simulink model "ex_mass_spring_damper_appdemo"  (R2024b)
settings: Solver=VariableStepAuto  StartTime=0.0  StopTime=10  MaxStep=0.025  RelTol=1e-3  AbsTol=1e-3  EnableMultiTasking=on
PreLoadFcn:
  | m = 3.600;     % kg
  | k = 400;    % N/m
  | b = 10;      % Ns/m
  | x0=1; %m
CloseFcn:
  | try,close(h1_MassSpringDamperInSimulinkAndSimscape),end
  | clear h1_MassSpringDamperInSimulinkAndSimscape
  | 
  | clear simlog_MassSpringDamperInSimulinkAndSimscape
  | clear logsout_MassSpringDamperInSimulinkAndSimscape
Description:
  | Mass-Spring-Damper in Simulink(R) and Simscape(TM)
settings Model: Creator=The MathWorks, Inc.  LastModifiedBy=The MathWorks, Inc.
settings SolverCC: AutoScaleAbsTol=off  AlgebraicLoopSolver=TrustRegion
settings DataIOCC: LimitDataPoints=on  SaveFormat=Array  SignalLoggingName=logsout_MassSpringDamperInSimulinkAndSimscape
settings OptimizationCC: LifeSpan=inf
settings DebuggingCC: SolverPrmCheckMsg=warning  UnconnectedInputMsg=warning  UnconnectedOutputMsg=warning  UnconnectedLineMsg=warning  AllowSymbolicDim=off  PregeneratedLibrarySubsystemCodeDiagnostic=none  SFUnexpectedBacktrackingDiag=warning  SFNoUnconditionalDefaultTransitionDiag=warning  SFExecutionAtInitializationDiag=none  ArithmeticOperatorsInVariantConditions=warning
settings HardwareCC: ProdBitPerPointer=32  ProdBitPerSizeT=32  ProdBitPerPtrDiffT=32  ProdLargestAtomicFloat=None  ProdIntDivRoundTo=Undefined  ProdEndianess=Unspecified  ProdWordSize=32  ProdHWDeviceType=32-bit Generic
settings ModelReferenceCC: EnableRefExpFcnMdlSchedulingChecks=on  PropagateSignalLabelsOutOfModel=off
settings SFSimCC: SimUseLocalCustomCode=off  CustomCodeUndefinedFunction=UseInterfaceOnly
settings RTWCC: RTWUseLocalCustomCode=off  GPUComputeCapability=3.5  DLArmComputeVersion=19.05
settings CodeAppCC: StateflowObjectComments=on
settings GRTTargetCC: TargetLangStandard=C89/C90 (ANSI)
settings ConfigComp: CovMetricSettings=dw  CovSaveCumulativeToWorkspaceVar=on  CovSaveSingleToWorkspaceVar=on  CovExternalEMLEnable=off  CovSFcnEnable=off
settings SimscapeCC: SimscapeLogType=all  SimscapeLogSimulationStatistics=on  SimscapeLogName=simlog_MassSpringDamperInSimulinkAndSimscape  SimscapeLogDataHistory=10000

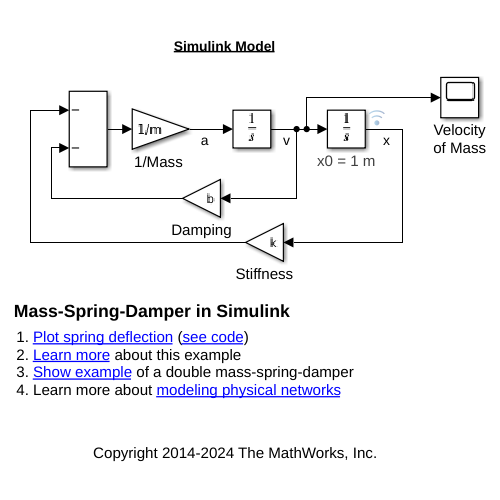
[thumbnail: Simulink's stored preview of the top-level diagram]
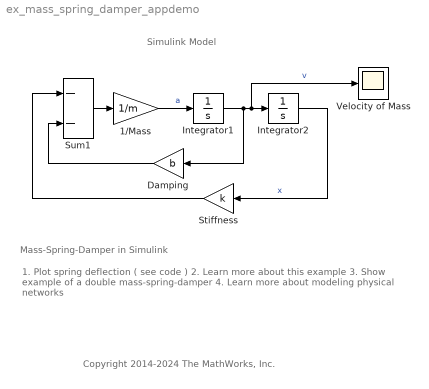
== system ex_mass_spring_damper_appdemo ==
  note: 1. Plot spring deflection ( see code )
      | 2. Learn more about this example
      | 3. Show example of a double mass-spring-damper
      | 4. Learn more about modeling physical networks
  note: Mass-Spring-Damper in Simulink
  note: Simulink Model
  note: Copyright 2014-2024 The MathWorks, Inc.
  "1/Mass " : Gain  Gain=1/m  SaturateOnIntegerOverflow=on  OutDataTypeStr=Inherit: Same as input  ParamDataTypeStr=Inherit: Same as input
  Damping : Gain  Gain=b  SaturateOnIntegerOverflow=on  OutDataTypeStr=Inherit: Same as input  ParamDataTypeStr=Inherit: Same as input
  Integrator1 : Integrator
  Integrator2 : Integrator  InitialCondition=1
      settings: AttributesFormatString=x0 = %<InitialCondition> m
  Stiffness : Gain  Gain=k  SaturateOnIntegerOverflow=on  OutDataTypeStr=Inherit: Same as input  ParamDataTypeStr=Inherit: Same as input
  Sum1 : Sum  Inputs=--  InputSameDT=on  SaturateOnIntegerOverflow=on  OutDataTypeStr=Inherit: Same as first input
  Velocity of Mass : Scope
  wires:
  "1/Mass "/1 -> Integrator1/1  "a"
  Sum1/1 -> "1/Mass "/1
  Damping/1 -> Sum1/2
  Stiffness/1 -> Sum1/1
  Integrator2/1 -> Stiffness/1  "x"
  Integrator1/1 -> Velocity of Mass/1, Integrator2/1, Damping/1  "v"
